simulink model "Simulink1"  (R2025b)
settings: Solver=ode45  StartTime=0.0  StopTime=Tsim  RelTol=1e-3
values from neighbouring files (symbols this model uses):
  c = c_min*3    [main.m]
  h1 = [0; 0; 0; 0]    [main.m]
  h2 = [1; 0; 0; 0]    [main.m]
  h3 = [0.5; 0; sqrt(3)/2; 0]    [main.m]
  K = inv(R)*B'*P_SVFB    [main.m]
  K_l = cl*K    [main.m]
  traj_choice = 2    [main.m]
  u_max = 2.5    [main.m]
  u_min = -2.5    [main.m]
  x1_0 = [3; 0; 1; 0]    [main.m]
  x2_0 = [-4; 0; 7; 0]    [main.m]
  x3_0 = [-2; 0; -4; 0]    [main.m]
settings Model: Creator=franc  LastModifiedBy=franc

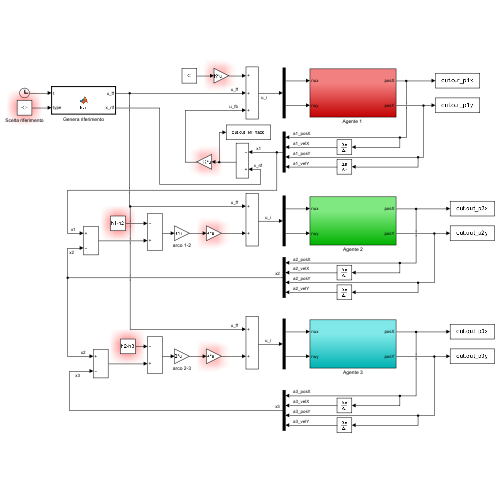
[thumbnail: Simulink's stored preview of the top-level diagram]
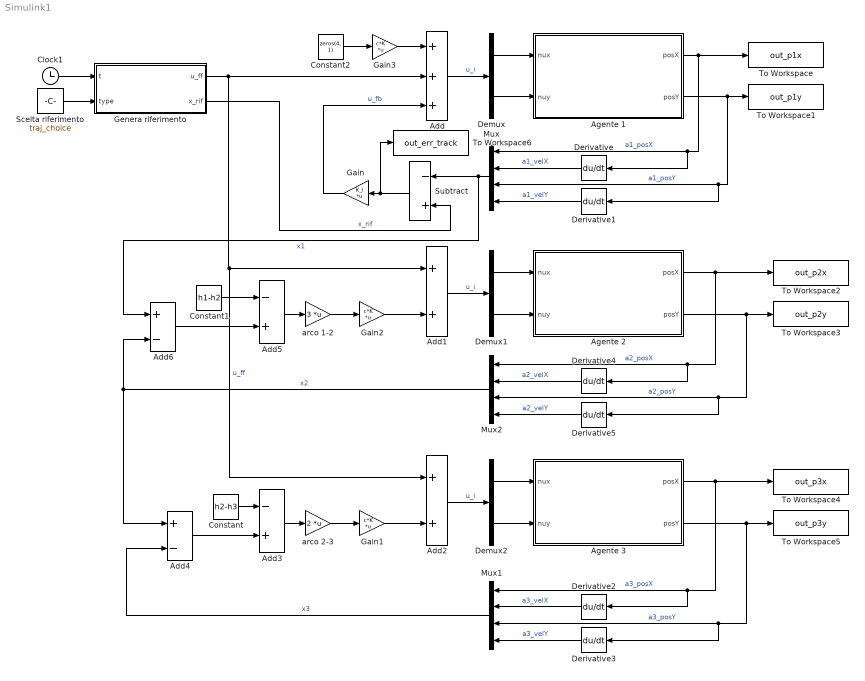
== system Simulink1 ==
  Add : Sum  Inputs=+++
  Add1 : Sum
  Add2 : Sum
  Add3 : Sum  Inputs=-+
  Add4 : Sum  Inputs=+-
  Add5 : Sum  Inputs=-+
  Add6 : Sum  Inputs=+-
  "Agente 1 " : Subsystem
  Agente 2 : Subsystem
  Agente 3 : Subsystem
  Clock1 : Clock
  Constant : Constant  Value=h2-h3
  Constant1 : Constant  Value=h1-h2
  Constant2 : Constant  Value=zeros(4, 1)
  Demux : Demux  Outputs=2
  Demux1 : Demux  Outputs=2
  Demux2 : Demux  Outputs=2
  Derivative{,1..5} (6 alike) : Derivative
  Gain : Gain  Gain=K_l  Multiplication=Matrix(K*u)
  Gain1 : Gain  Gain=c*K  Multiplication=Matrix(K*u)
  Gain2 : Gain  Gain=c*K  Multiplication=Matrix(K*u)
  Gain3 : Gain  Gain=c*K  Multiplication=Matrix(K*u)
  Genera riferimento : MATLAB Function  TreatAsAtomicUnit=on
  Mux : Mux
  Mux1 : Mux
  Mux2 : Mux
  Scelta riferimento : Constant  Value=traj_choice
  Subtract : Sum  Inputs=-+
  To Workspace : ToWorkspace  VariableName=out_p1x  SampleTime=-1
  To Workspace1 : ToWorkspace  VariableName=out_p1y  SampleTime=-1
  To Workspace2 : ToWorkspace  VariableName=out_p2x  SampleTime=-1
  To Workspace3 : ToWorkspace  VariableName=out_p2y  SampleTime=-1
  To Workspace4 : ToWorkspace  VariableName=out_p3x  SampleTime=-1
  To Workspace5 : ToWorkspace  VariableName=out_p3y  SampleTime=-1
  To Workspace6 : ToWorkspace  VariableName=out_err_track  SampleTime=-1
  arco 1-2 : Gain  Gain=3  Multiplication=Matrix(K*u)
  arco 2-3 : Gain  Gain=2  Multiplication=Matrix(K*u)
  wires:
  Derivative3/1 -> Mux1/4  "a3_velY"
  Demux/1 -> "Agente 1 "/1(nux)
  Demux1/2 -> Agente 2/2(nuy)
  Constant/1 -> Add3/1
  Agente 3/2(posY) -> To Workspace5/1, Mux1/3, Derivative3/1  "a3_posY"
  arco 1-2/1 -> Gain2/1
  Derivative/1 -> Mux/2  "a1_velX"
  Mux1/1 -> Add4/2  "x3"
  Add4/1 -> Add3/2
  Gain3/1 -> Add/1
  Derivative5/1 -> Mux2/4  "a2_velY"
  Gain2/1 -> Add1/2
  Demux2/2 -> Agente 3/2(nuy)
  Derivative2/1 -> Mux1/2  "a3_velX"
  Gain/1 -> Add/3  "u_fb"
  Add5/1 -> arco 1-2/1
  Gain1/1 -> Add2/2
  Subtract/1 -> To Workspace6/1, Gain/1
  arco 2-3/1 -> Gain1/1
  Add1/1 -> Demux1/1  "u_i"
  Demux2/1 -> Agente 3/1(nux)
  Add6/1 -> Add5/2
  Add2/1 -> Demux2/1  "u_i"
  Genera riferimento/1(u_ff) -> Add2/1, Add1/1, Add/2  "u_ff"
  Genera riferimento/2(x_rif) -> Subtract/2  "x_rif"
  Derivative4/1 -> Mux2/2  "a2_velX"
  Demux/2 -> "Agente 1 "/2(nuy)
  "Agente 1 "/2(posY) -> To Workspace1/1, Derivative1/1, Mux/3  "a1_posY"
  Mux2/1 -> Add6/2, Add4/1  "x2"
  Constant1/1 -> Add5/1
  Derivative1/1 -> Mux/4  "a1_velY"
  "Agente 1 "/1(posX) -> To Workspace/1, Mux/1, Derivative/1  "a1_posX"
  Agente 3/1(posX) -> To Workspace4/1, Mux1/1, Derivative2/1  "a3_posX"
  Agente 2/2(posY) -> To Workspace3/1, Mux2/3, Derivative5/1  "a2_posY"
  Agente 2/1(posX) -> To Workspace2/1, Mux2/1, Derivative4/1  "a2_posX"
  Constant2/1 -> Gain3/1
  Add3/1 -> arco 2-3/1
  Demux1/1 -> Agente 2/1(nux)
  Mux/1 -> Add6/1, Subtract/1  "x1"
  Scelta riferimento/1 -> Genera riferimento/2(type)
  Clock1/1 -> Genera riferimento/1(t)
  Add/1 -> Demux/1  "u_i"

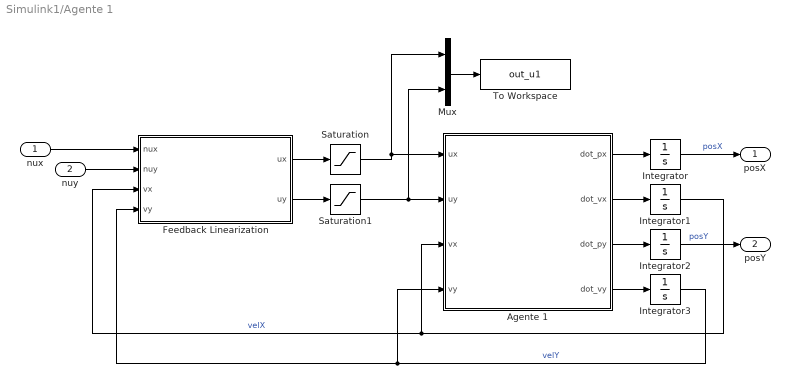
== system Simulink1/Agente 1  ==
  nux : Inport
  nuy : Inport  Port=2
  Agente 1 : MATLAB Function  TreatAsAtomicUnit=on
  Feedback Linearization : MATLAB Function  TreatAsAtomicUnit=on
  Integrator : Integrator  InitialCondition=x1_0(1)
  Integrator1 : Integrator  InitialCondition=x1_0(2)
  Integrator2 : Integrator  InitialCondition=x1_0(3)
  Integrator3 : Integrator  InitialCondition=x1_0(4)
  Mux : Mux  Inputs=2
  Saturation : Saturate  UpperLimit=u_max  LowerLimit=u_min
  Saturation1 : Saturate  UpperLimit=u_max  LowerLimit=u_min
  To Workspace : ToWorkspace  VariableName=out_u1  SampleTime=-1
  posX : Outport
  posY : Outport  Port=2
  wires:
  Agente 1/3(dot_py) -> Integrator2/1
  Integrator1/1 -> Feedback Linearization/3(vx), Agente 1/3(vx)  "velX"
  Feedback Linearization/1(ux) -> Saturation/1
  Feedback Linearization/2(uy) -> Saturation1/1
  Integrator3/1 -> Feedback Linearization/4(vy), Agente 1/4(vy)  "velY"
  Integrator/1 -> posX/1  "posX"
  Agente 1/1(dot_px) -> Integrator/1
  Agente 1/2(dot_vx) -> Integrator1/1
  Agente 1/4(dot_vy) -> Integrator3/1
  nux/1 -> Feedback Linearization/1(nux)
  Integrator2/1 -> posY/1  "posY"
  nuy/1 -> Feedback Linearization/2(nuy)
  Mux/1 -> To Workspace/1
  Saturation/1 -> Agente 1/1(ux), Mux/1
  Saturation1/1 -> Agente 1/2(uy), Mux/2

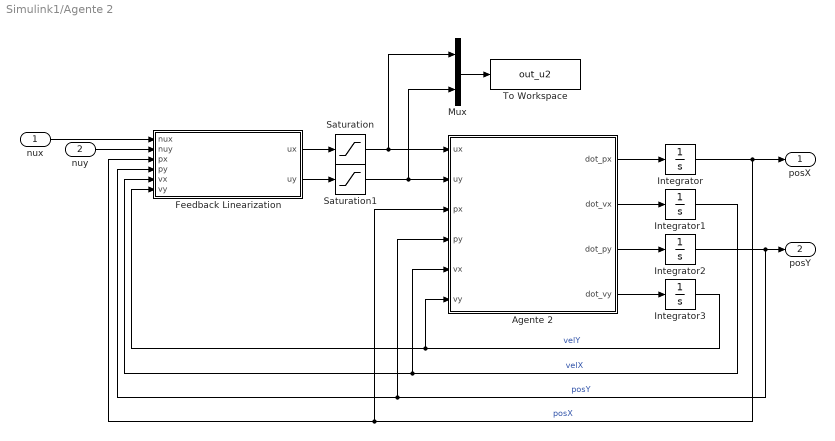
== system Simulink1/Agente 2 ==
  nux : Inport
  nuy : Inport  Port=2
  Agente 2 : MATLAB Function  TreatAsAtomicUnit=on
  Feedback Linearization : MATLAB Function  TreatAsAtomicUnit=on
  Integrator : Integrator  InitialCondition=x2_0(1)
  Integrator1 : Integrator  InitialCondition=x2_0(2)
  Integrator2 : Integrator  InitialCondition=x2_0(3)
  Integrator3 : Integrator  InitialCondition=x2_0(4)
  Mux : Mux  Inputs=2
  Saturation : Saturate  UpperLimit=u_max  LowerLimit=u_min
  Saturation1 : Saturate  UpperLimit=u_max  LowerLimit=u_min
  To Workspace : ToWorkspace  VariableName=out_u2  SampleTime=-1
  posX : Outport
  posY : Outport  Port=2
  wires:
  Agente 2/3(dot_py) -> Integrator2/1
  Feedback Linearization/1(ux) -> Saturation/1
  Feedback Linearization/2(uy) -> Saturation1/1
  Integrator/1 -> Agente 2/3(px), Feedback Linearization/3(px), posX/1  "posX"
  Agente 2/1(dot_px) -> Integrator/1
  Agente 2/2(dot_vx) -> Integrator1/1
  Agente 2/4(dot_vy) -> Integrator3/1
  nux/1 -> Feedback Linearization/1(nux)
  Integrator2/1 -> Agente 2/4(py), Feedback Linearization/4(py), posY/1  "posY"
  nuy/1 -> Feedback Linearization/2(nuy)
  Integrator3/1 -> Agente 2/6(vy), Feedback Linearization/6(vy)  "velY"
  Integrator1/1 -> Agente 2/5(vx), Feedback Linearization/5(vx)  "velX"
  Mux/1 -> To Workspace/1
  Saturation/1 -> Mux/1, Agente 2/1(ux)
  Saturation1/1 -> Mux/2, Agente 2/2(uy)

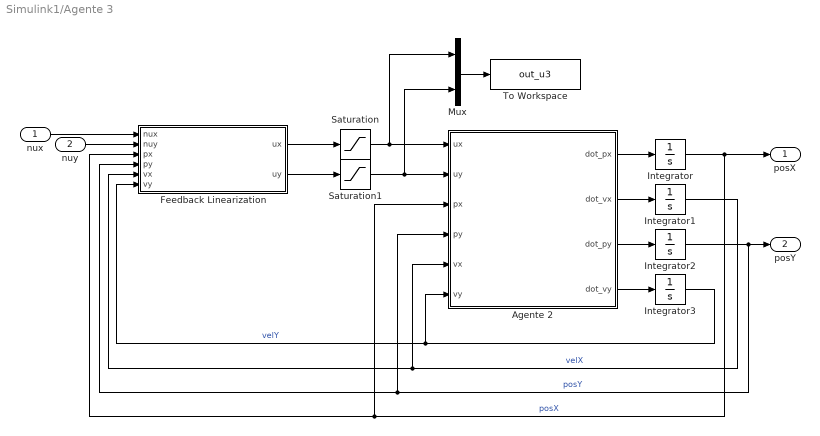
== system Simulink1/Agente 3 ==
  nux : Inport
  nuy : Inport  Port=2
  Agente 2 : MATLAB Function  TreatAsAtomicUnit=on
  Feedback Linearization : MATLAB Function  TreatAsAtomicUnit=on
  Integrator : Integrator  InitialCondition=x3_0(1)
  Integrator1 : Integrator  InitialCondition=x3_0(2)
  Integrator2 : Integrator  InitialCondition=x3_0(3)
  Integrator3 : Integrator  InitialCondition=x3_0(4)
  Mux : Mux  Inputs=2
  Saturation : Saturate  UpperLimit=u_max  LowerLimit=u_min
  Saturation1 : Saturate  UpperLimit=u_max  LowerLimit=u_min
  To Workspace : ToWorkspace  VariableName=out_u3  SampleTime=-1
  posX : Outport
  posY : Outport  Port=2
  wires:
  Agente 2/3(dot_py) -> Integrator2/1
  Feedback Linearization/1(ux) -> Saturation/1
  Feedback Linearization/2(uy) -> Saturation1/1
  Integrator/1 -> posX/1, Agente 2/3(px), Feedback Linearization/3(px)  "posX"
  Agente 2/1(dot_px) -> Integrator/1
  Agente 2/2(dot_vx) -> Integrator1/1
  Agente 2/4(dot_vy) -> Integrator3/1
  nux/1 -> Feedback Linearization/1(nux)
  Integrator2/1 -> Agente 2/4(py), Feedback Linearization/4(py), posY/1  "posY"
  nuy/1 -> Feedback Linearization/2(nuy)
  Integrator3/1 -> Agente 2/6(vy), Feedback Linearization/6(vy)  "velY"
  Integrator1/1 -> Agente 2/5(vx), Feedback Linearization/5(vx)  "velX"
  Mux/1 -> To Workspace/1
  Saturation/1 -> Mux/1, Agente 2/1(ux)
  Saturation1/1 -> Mux/2, Agente 2/2(uy)

== matlab function Simulink1/Agente 1 /Feedback Linearization ==
  data: nux input; ux output; nuy input; vx input; vy input; uy output
function [ux, uy] = agent1_fl(nux, nuy, vx, vy)
    phi_x = -0.35*vx - 0.08*vx*abs(vx);
    phi_y = -0.45*vy - 0.10*vy*abs(vy);
    % B = diag([1/1.2, 1/1.2]) -> det(B) != 0
    ux = 1.2 * (nux - phi_x);
    uy = 1.2 * (nuy - phi_y);
end

== matlab function Simulink1/Agente 1 /Agente 1 ==
  data: ux input; dot_px output; uy input; vx input; vy input; dot_vx output; dot_py output; dot_vy output
function [dot_px, dot_vx, dot_py, dot_vy] = agent1_dynamics(ux, uy, vx, vy)
    % Equazioni differenziali REALI del robot -> non lineari !!
    dot_px = vx;
    dot_vx = -0.35*vx - 0.08*vx*abs(vx) + (1/1.2)*ux;
    
    dot_py = vy;
    dot_vy = -0.45*vy - 0.10*vy*abs(vy) + (1/1.2)*uy;
end

== matlab function Simulink1/Agente 2/Agente 2 ==
  data: ux input; dot_px output; uy input; px input; py input; vx input; vy input; dot_vx output; dot_py output; dot_vy output
function [dot_px, dot_vx, dot_py, dot_vy] = fcn(ux, uy, px, py, vx, vy)
    % Dinamica reale dell'Agente 2 -> non lineare !!
    dot_px = vx;
    dot_vx = -0.40 * vx + (1 / (1 + 0.25 * sin(px)^2)) * ux;
    
    dot_py = vy;
    dot_vy = -0.55 * vy + (1 / (1 + 0.30 * cos(py)^2)) * uy;
end

== matlab function Simulink1/Agente 2/Feedback Linearization ==
  data: nux input; ux output; nuy input; px input; py input; vx input; vy input; uy output
function [ux, uy] = fcn(nux, nuy, px, py, vx, vy)
    phi_x = -0.40 * vx;
    phi_y = -0.55 * vy;
   
    ux = (1 + 0.25 * sin(px)^2) * (nux - phi_x);
    uy = (1 + 0.30 * cos(py)^2) * (nuy - phi_y);
end

== matlab function Simulink1/Agente 3/Agente 2 ==
  data: ux input; dot_px output; uy input; px input; py input; vx input; vy input; dot_vx output; dot_py output; dot_vy output
function [dot_px, dot_vx, dot_py, dot_vy] = fcn(ux, uy, px, py, vx, vy)
    u = [ux; uy];

    dot_px = vx;
    dot_py = vy;
    
    phi = [ -0.30*vx + 0.15*sin(py)*vy;
            -0.35*vy + 0.15*cos(px)*vx ];
            
    B = [ 1 + 0.20*cos(py)^2,  0.08*sin(px);
          0.08*sin(py),         1 + 0.20*sin(px)^2 ];
          
    dot_v = phi + B * u;
    
    dot_vx = dot_v(1);
    dot_vy = dot_v(2);
end

== matlab function Simulink1/Agente 3/Feedback Linearization ==
  data: nux input; ux output; nuy input; px input; py input; vx input; vy input; uy output
function [ux, uy] = fcn(nux, nuy, px, py, vx, vy)
    % Vettore di ingresso virtuale
    nu = [nux; nuy];

    phi = [ -0.30*vx + 0.15*sin(py)*vy;
            -0.35*vy + 0.15*cos(px)*vx ];
            
    % B sempre invertibile
    B = [ 1 + 0.20*cos(py)^2,  0.08*sin(px);
          0.08*sin(py),         1 + 0.20*sin(px)^2 ];
          
    % u -> vettore di ingressi fisici
    u = B \ (nu - phi);
    
    ux = u(1);
    uy = u(2);
end

== matlab function Simulink1/Genera riferimento ==
  data: t input; u_ff output; x_rif output; type input
function [u_ff, x_rif] = fcn(t,type)
    % ----- Riferimento velocità costante -----
    r0 = [0; 0];
    v_ref_const = [0.5; 0.5]; 
    % ----- Riferimento circolare -----
    rc = [0; 5];              
    Rc = 5;           
    omega_c = 0.5;    
    % ----- Riferimento sinusoidale -----
    v_x_sin = 0.5;           
    A_sin = 3;        
    omega_sin = 1; 

    % --- 1. CALCOLO DELLA TRAIETTORIA DI RIFERIMENTO ---
    if type == 1            % ----- Riferimento velocità costante -----
        p_rif = r0 + v_ref_const * t;
        v_rif = v_ref_const; 
        u_ff = [0;0];
    elseif type == 2        % ----- Riferimento circolare -----
        p_rif = rc + Rc * [cos(omega_c*t); sin(omega_c*t)];
        v_rif = Rc * omega_c * [-sin(omega_c*t); cos(omega_c*t)];
        u_ff = -Rc * omega_c^2 * [cos(omega_c*t); sin(omega_c*t)];
    else                    % ----- Riferimento sinusoidale -----
        p_rif = [r0(1) + v_x_sin * t; r0(2) + A_sin * sin(omega_sin * t)];
        v_rif = [v_x_sin; A_sin * omega_sin * cos(omega_sin * t)];
        u_ff = [0; -A_sin * omega_sin^2 * sin(omega_sin * t)];
    end
    
    % --- 2. ASSEGNAZIONE DELLE USCITE DEL BLOCCO ---

    % VETTORE DI STATO RIFERIMENTO (vettore colonna 4x1)
    x_rif = [p_rif(1); 
             v_rif(1); 
             p_rif(2); 
             v_rif(2)];
end
